simulink model "SolvingDE1"  (R2020b)
settings: Solver=VariableStepAuto  StartTime=0.0  StopTime=10.0  RelTol=1e-3
settings Model: Creator=riwakaram  LastModifiedBy=riwakaram

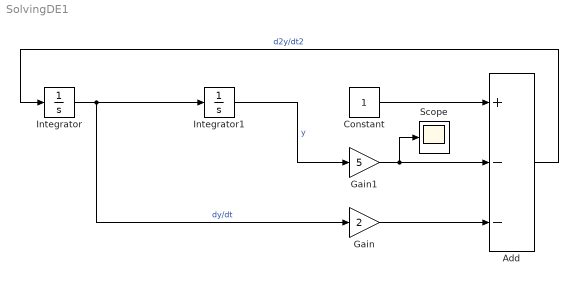
== system SolvingDE1 ==
  Add : Sum  Inputs=+--
  Constant : Constant
  Gain : Gain  Gain=2
  Gain1 : Gain  Gain=5
  Integrator : Integrator
  Integrator1 : Integrator
  Scope : Scope
  wires:
  Integrator/1 -> Gain/1, Integrator1/1  "dy/dt"
  Constant/1 -> Add/1
  Integrator1/1 -> Gain1/1  "y"
  Gain/1 -> Add/3
  Add/1 -> Integrator/1  "d2y/dt2"
  Gain1/1 -> Add/2, Scope/1
